simulink model "encoder"  (R2023a)
settings: Solver=FixedStepDiscrete  StartTime=0.0  StopTime=0.02  FixedStep=0.0005  RelTol=1e-3
libraries: simulink x2
settings Model: Creator=Nacho Andrade  LastModifiedBy=Nacho Andrade

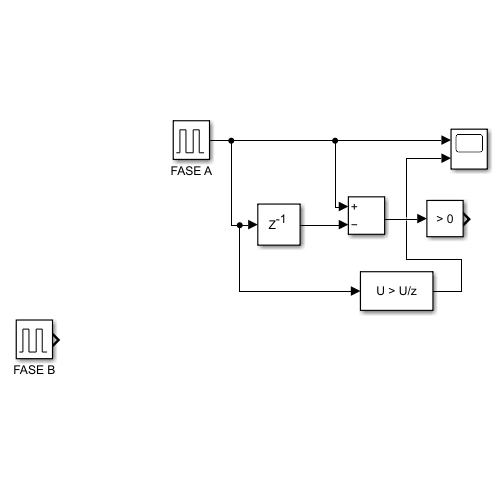
[thumbnail: Simulink's stored preview of the top-level diagram]
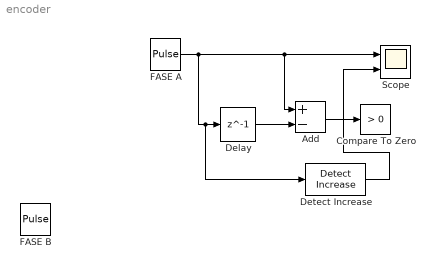
== system encoder ==
  Add : Sum  Inputs=+-
  Compare To Zero : simulink/Logic and Bit Operations/Compare To Zero  relop=>  OutDataTypeStr=boolean
  Delay : Delay  DelayLength=1
  Detect Increase : simulink/Logic and Bit Operations/Detect Increase  vinit=0.0  OutDataTypeStr=boolean
      settings: LibrarySourceBlock=|
      | hdlsllib/Logic and Bit
      | Operations/Detect
      | Increase
  "FASE A " : DiscretePulseGenerator  PulseType=Time based  Amplitude=5  Period=0.002  PulseWidth=50
  FASE B : DiscretePulseGenerator  PulseType=Time based  Amplitude=5  Period=0.002  PulseWidth=50  PhaseDelay=.0005
  Scope : Scope  NumInputPorts=2
  wires:
  "FASE A "/1 -> Scope/1, Add/1, Detect Increase/1, Delay/1
  Delay/1 -> Add/2
  Add/1 -> Compare To Zero/1
  Detect Increase/1 -> Scope/2
